simulink model "upper_limit_sliding_mode_comp_sat_sign"  (R2019b)
settings: Solver=VariableStepAuto  StartTime=0.0  StopTime=10  RelTol=1e-3
settings Model: Creator=Alien  LastModifiedBy=Alien
settings SolverCC: ZeroCrossAlgorithm=Adaptive
settings DebuggingCC: IgnoredZcDiagnostic=none

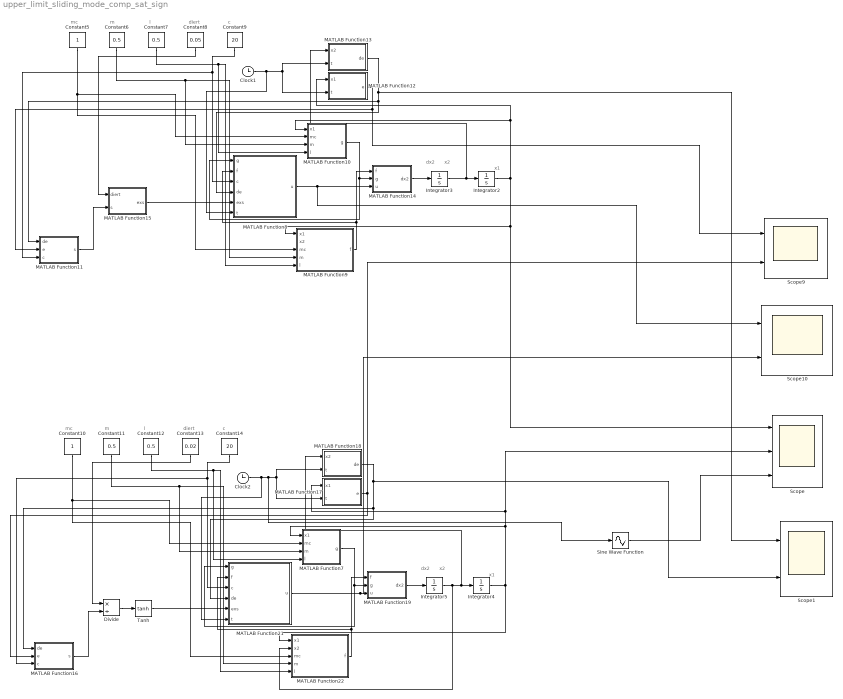
== system upper_limit_sliding_mode_comp_sat_sign ==
  note: diert
  note: l
  note: m
  note: x2
  note: x1
  note: dx2
  note: c
  note: mc
  note: x1
  note: dx2
  note: x2
  note: m
  note: diert
  note: mc
  note: l
  note: c
  Clock1 : Clock
  Clock2 : Clock
  Constant10 : Constant
  Constant{6..7,11..12} (4 alike) : Constant  Value=0.5
  Constant13 : Constant  Value=0.02
  Constant14 : Constant  Value=20
  Constant5 : Constant
  Constant8 : Constant  Value=0.05
  Constant9 : Constant  Value=20
  Divide : Product  Inputs=*/
  Integrator2 : Integrator
  Integrator3 : Integrator  InitialCondition=pi/60
  Integrator4 : Integrator
  Integrator5 : Integrator  InitialCondition=pi/60
  MATLAB Function10 : MATLAB Function  TreatAsAtomicUnit=on
  MATLAB Function11 : MATLAB Function  TreatAsAtomicUnit=on
  MATLAB Function12 : MATLAB Function  TreatAsAtomicUnit=on
  MATLAB Function13 : MATLAB Function  TreatAsAtomicUnit=on
  MATLAB Function14 : MATLAB Function  TreatAsAtomicUnit=on
  MATLAB Function15 : MATLAB Function  TreatAsAtomicUnit=on
  MATLAB Function16 : MATLAB Function  TreatAsAtomicUnit=on
  MATLAB Function17 : MATLAB Function  TreatAsAtomicUnit=on
  MATLAB Function18 : MATLAB Function  TreatAsAtomicUnit=on
  MATLAB Function19 : MATLAB Function  TreatAsAtomicUnit=on
  MATLAB Function21 : MATLAB Function  TreatAsAtomicUnit=on
  MATLAB Function22 : MATLAB Function  TreatAsAtomicUnit=on
  MATLAB Function7 : MATLAB Function  TreatAsAtomicUnit=on
  MATLAB Function8 : MATLAB Function  TreatAsAtomicUnit=on
  MATLAB Function9 : MATLAB Function  TreatAsAtomicUnit=on
  Scope : Scope  NumInputPorts=3
  Scope1 : Scope  NumInputPorts=2
  Scope10 : Scope  NumInputPorts=2
  Scope9 : Scope  NumInputPorts=2
  Sine Wave Function : Sin  TimeSource=Use external signal  Amplitude=0.1  SampleTime=0
  Tanh : Trigonometry  Operator=tanh
  wires:
  MATLAB Function10/1(g) -> MATLAB Function8/1(g), MATLAB Function14/2(g)
  Constant8/1 -> MATLAB Function15/1(diert)
  MATLAB Function11/1(s) -> MATLAB Function15/2(s)
  MATLAB Function13/1(de) -> Scope1/1, MATLAB Function11/1(de), MATLAB Function8/4(de)
  Clock1/1 -> MATLAB Function8/6(t), MATLAB Function12/2(t), MATLAB Function13/2(t)
  Constant7/1 -> MATLAB Function10/4(l), MATLAB Function9/5(l)
  Constant6/1 -> MATLAB Function10/3(m), MATLAB Function9/4(m)
  MATLAB Function12/1(e) -> MATLAB Function11/2(e), Scope9/1
  Integrator3/1 -> MATLAB Function13/1(x2), Integrator2/1
  MATLAB Function14/1(dx2) -> Integrator3/1
  Constant9/1 -> MATLAB Function11/3(c), MATLAB Function8/3(c)
  MATLAB Function9/1(f) -> MATLAB Function14/1(f), MATLAB Function8/2(f)
  Integrator2/1 -> Scope/1, MATLAB Function9/1(x1), MATLAB Function12/1(x1), MATLAB Function10/1(x1)
  Constant5/1 -> MATLAB Function10/2(mc), MATLAB Function9/3(mc)
  MATLAB Function8/1(u) -> Scope10/1, MATLAB Function14/3(u)
  MATLAB Function15/1(exs) -> MATLAB Function8/5(exs)
  Constant12/1 -> MATLAB Function7/4(l), MATLAB Function22/5(l)
  Clock2/1 -> MATLAB Function21/6(t), Sine Wave Function/1, MATLAB Function17/2(t), MATLAB Function18/2(t)
  MATLAB Function7/1(g) -> MATLAB Function21/1(g), MATLAB Function19/2(g)
  MATLAB Function21/1(u) -> Scope10/2, MATLAB Function19/3(u)
  Constant10/1 -> MATLAB Function7/2(mc), MATLAB Function22/3(mc)
  MATLAB Function17/1(e) -> Scope9/2, MATLAB Function16/2(e)
  Constant14/1 -> MATLAB Function16/3(c), MATLAB Function21/3(c)
  MATLAB Function18/1(de) -> Scope1/2, MATLAB Function16/1(de), MATLAB Function21/4(de)
  Integrator5/1 -> MATLAB Function22/2(x2), MATLAB Function18/1(x2), Integrator4/1
  Constant13/1 -> Divide/1
  Integrator4/1 -> MATLAB Function22/1(x1), Scope/2, MATLAB Function17/1(x1), MATLAB Function7/1(x1)
  MATLAB Function22/1(f) -> MATLAB Function19/1(f), MATLAB Function21/2(f)
  MATLAB Function19/1(dx2) -> Integrator5/1
  MATLAB Function16/1(s) -> Divide/2
  Constant11/1 -> MATLAB Function7/3(m), MATLAB Function22/4(m)
  Divide/1 -> Tanh/1
  Tanh/1 -> MATLAB Function21/5(exs)
  Sine Wave Function/1 -> Scope/3

== matlab function upper_limit_sliding_mode_comp_sat_sign/MATLAB Function16 ==
  data: de input; s output; e input; c input
function s = fcn(de, e, c)
s = de + c*e;

== matlab function upper_limit_sliding_mode_comp_sat_sign/MATLAB Function10 ==
  data: x1 input; g output; mc input; m input; l input
function g = fcn(x1, mc, m, l)
g = (cos(x1)/(mc + m))/(l*(4/3 - m*((cos(x1))^2)/(mc +m)));

== matlab function upper_limit_sliding_mode_comp_sat_sign/MATLAB Function11 ==
  data: de input; s output; e input; c input
function s = fcn(de, e, c)
s = de + c*e;

== matlab function upper_limit_sliding_mode_comp_sat_sign/MATLAB Function12 ==
  data: x1 input; e output; t input
function e = fcn(x1, t)
e = 0.1*sin(t) - x1;

== matlab function upper_limit_sliding_mode_comp_sat_sign/MATLAB Function13 ==
  data: x2 input; de output; t input
function de = fcn(x2, t)
de = 0.1*cos(t) - x2;

== matlab function upper_limit_sliding_mode_comp_sat_sign/MATLAB Function14 ==
  data: f input; g input; u input; dx2 output
function dx2 = fcn(f, g, u)
dx2 = f + g*u;

== matlab function upper_limit_sliding_mode_comp_sat_sign/MATLAB Function15 ==
  data: diert input; exs output; s input
function exs = fcn(diert, s)
if s > diert
    exs = 1;
elseif s < -diert
    exs = -1;
else
    exs = 1/diert*s;
end

== matlab function upper_limit_sliding_mode_comp_sat_sign/MATLAB Function8 ==
  data: g input; u output; f input; c input; de input; exs input; t input
function u = fcn(g, f, c, de, exs, t)
nta = 0.2;
ddx1d = -0.1 * sin(t);
u = 1/g*(ddx1d - f + c * de + nta * exs);

== matlab function upper_limit_sliding_mode_comp_sat_sign/MATLAB Function9 ==
  data: x1 input; f output; x2 input; mc input; m input; l input
function f = fcn(x1, x2, mc, m, l)
g = 9.8;
f = (g*sin(x1) - m*l*((x2)^2)*cos(x1)*sin(x1)/(mc +m))/(l*(4/3 - m * ((cos(x1))^2)/(mc + m)));

== matlab function upper_limit_sliding_mode_comp_sat_sign/MATLAB Function17 ==
  data: x1 input; e output; t input
function e = fcn(x1, t)
e = 0.1*sin(t) - x1;

== matlab function upper_limit_sliding_mode_comp_sat_sign/MATLAB Function18 ==
  data: x2 input; de output; t input
function de = fcn(x2, t)
de = 0.1*cos(t) - x2;

== matlab function upper_limit_sliding_mode_comp_sat_sign/MATLAB Function19 ==
  data: f input; g input; u input; dx2 output
function dx2 = fcn(f, g, u)
dx2 = f + g*u;

== matlab function upper_limit_sliding_mode_comp_sat_sign/MATLAB Function21 ==
  data: g input; u output; f input; c input; de input; exs input; t input
function u = fcn(g, f, c, de, exs, t)
nta = 0.2;
ddx1d = -0.1 * sin(t);
u = 1/g*(ddx1d - f + c * de + nta * exs);

== matlab function upper_limit_sliding_mode_comp_sat_sign/MATLAB Function22 ==
  data: x1 input; f output; x2 input; mc input; m input; l input
function f = fcn(x1, x2, mc, m, l)
g = 9.8;
f = (g*sin(x1) - m*l*((x2)^2)*cos(x1)*sin(x1)/(mc +m))/(l*(4/3 - m * ((cos(x1))^2)/(mc + m)));

== matlab function upper_limit_sliding_mode_comp_sat_sign/MATLAB Function7 ==
  data: x1 input; g output; mc input; m input; l input
function g = fcn(x1, mc, m, l)
g = (cos(x1)/(mc + m))/(l*(4/3 - m*((cos(x1))^2)/(mc +m)));
